simulink model "Simulinkk_Ex6"  (R2024b)
settings: Solver=VariableStepAuto  StartTime=0.0  StopTime=10.0  RelTol=1e-3
values from neighbouring files (symbols this model uses):
  c = c2    (= 0.5)    [Ex6.m]    (also in Ex6_d.m = 1)
  k = k0    (= 10)    [Ex6.m]    (also in Ex6_d.m = 30)
  m = 3    [Ex6.m]    (also in Ex6_d.m)
settings Model: Creator=eduardo  LastModifiedBy=eduardo

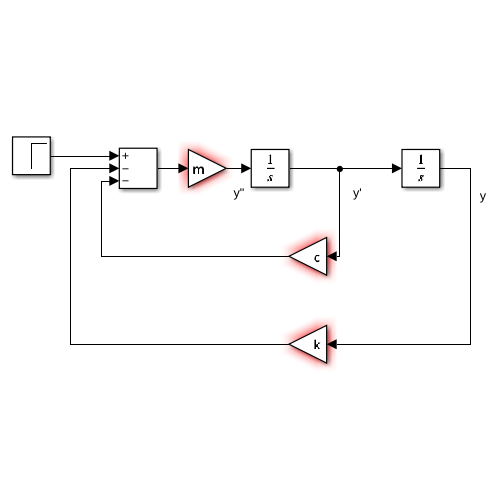
[thumbnail: Simulink's stored preview of the top-level diagram]
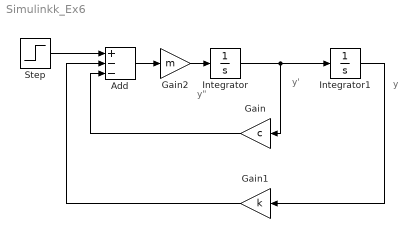
== system Simulinkk_Ex6 ==
  note: y
  note: y'
  note: y"
  Add : Sum  Inputs=+--
  Gain : Gain  Gain=c
  Gain1 : Gain  Gain=k
  Gain2 : Gain  Gain=m
  Integrator : Integrator
  Integrator1 : Integrator
  Step : Step  After=3  SampleTime=0
  wires:
  Integrator/1 -> Gain/1, Integrator1/1
  Integrator1/1 -> Gain1/1
  Gain/1 -> Add/3
  Gain1/1 -> Add/2
  Step/1 -> Add/1
  Add/1 -> Gain2/1
  Gain2/1 -> Integrator/1
